simulink model "LQG_tw_v5"  (R2019a)
settings: Solver=FixedStepAuto  StartTime=0.0  StopTime=20  FixedStep=0.01  RelTol=1e-3
undefined symbols (not defined in the file): K
libraries: simulink x3, simulink_extras x2
settings Model: Creator=chute  LastModifiedBy=chute
settings DataIOCC: ReturnWorkspaceOutputs=off

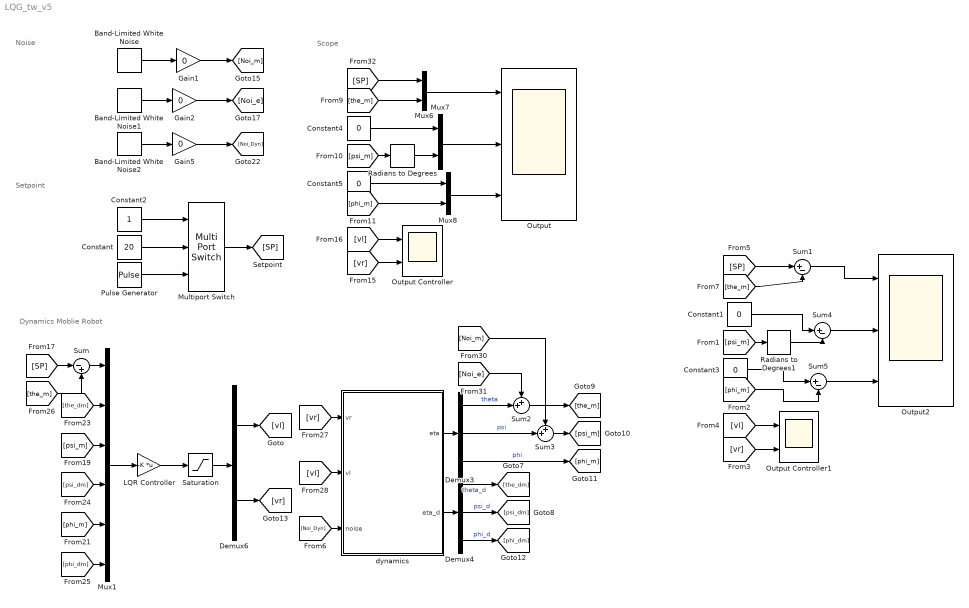
== system LQG_tw_v5 ==
  note: Noise
  note: Scope
  note: Setpoint
  note: Dynamics Moblie Robot
  Band-Limited White Noise : simulink/Sources/Band-Limited White Noise  Cov=[0.0001]  Ts=0.1  seed=[23341]
  Band-Limited White Noise1 : simulink/Sources/Band-Limited White Noise  Cov=[0.0001]  Ts=0.1  seed=[23341]
  Band-Limited White Noise2 : simulink/Sources/Band-Limited White Noise  Cov=[0.0001]  Ts=0.1  seed=[23341]
  Constant : Constant  Value=20
  Constant{1,3..5} (4 alike) : Constant  Value=0
  Constant2 : Constant
  Demux3 : Demux  Outputs=3
  Demux4 : Demux  Outputs=3
  Demux6 : Demux  Outputs=2
  Gain1 : Gain  Gain=0
  Gain2 : Gain  Gain=0
  Gain5 : Gain  Gain=0
  LQR Controller : Gain  Gain=-K  Multiplication=Matrix(K*u) (u vector)
  Multiport Switch : MultiPortSwitch  Inputs=2
  Mux1 : Mux  Inputs=6
  Mux6 : Mux  Inputs=2
  Mux7 : Mux  Inputs=2
  Mux8 : Mux  Inputs=2
  Output : Scope  NumInputPorts=3
  Output Controller : Scope  NumInputPorts=2
  Output Controller1 : Scope  NumInputPorts=2
  Output2 : Scope  NumInputPorts=3
  Pulse Generator : DiscretePulseGenerator  PulseType=Time based  Amplitude=20  Period=10  PulseWidth=50
  Radians to Degrees : simulink_extras/Transformations/Radians to Degrees
  Radians to Degrees1 : simulink_extras/Transformations/Radians to Degrees
  Saturation : Saturate  UpperLimit=12  LowerLimit=-12
  Sum : Sum  Inputs=|-+
  Sum1 : Sum  Inputs=|+-
  Sum2 : Sum  Inputs=++|
  Sum3 : Sum  Inputs=++|
  Sum4 : Sum  Inputs=|+-
  Sum5 : Sum  Inputs=|+-
  dynamics : Subsystem
  wires:
  dynamics/1(eta) -> Demux3/1
  Demux4/1 -> [the_dm]  "theta_d"
  dynamics/2(eta_d) -> Demux4/1
  Demux4/3 -> [phi_dm]  "phi_d"
  Demux4/2 -> [psi_dm]  "psi_d"
  Demux6/1 -> [vl]
  LQR Controller/1 -> Saturation/1
  Mux1/1 -> LQR Controller/1
  Sum/1 -> Mux1/1
  Multiport Switch/1 -> [SP]
  Constant/1 -> Multiport Switch/2
  Constant2/1 -> Multiport Switch/1
  [phi_m] -> Mux1/5
  [psi_m] -> Mux1/3
  [the_dm] -> Mux1/2
  [psi_dm] -> Mux1/4
  [phi_dm] -> Mux1/6
  Band-Limited White Noise/1 -> Gain1/1
  Demux3/3 -> [phi_m]  "phi"
  Sum3/1 -> [psi_m]
  Demux3/2 -> Sum3/2  "psi"
  Demux3/1 -> Sum2/2  "theta"
  Band-Limited White Noise1/1 -> Gain2/1
  [the_m] -> Sum/2
  [vl] -> dynamics/2("vl ")
  [vr] -> dynamics/1(vr)
  Gain1/1 -> [Noi_m]
  Gain2/1 -> [Noi_e]
  [Noi_m] -> Sum3/1
  [Noi_e] -> Sum2/1
  Mux8/1 -> Output/3
  Mux7/1 -> Output/2
  Mux6/1 -> Output/1
  [the_m] -> Mux6/2
  [SP] -> Mux6/1
  [psi_m] -> Radians to Degrees/1
  Constant4/1 -> Mux7/1
  [phi_m] -> Mux8/2
  Constant5/1 -> Mux8/1
  Sum2/1 -> [the_m]
  Demux6/2 -> [vr]
  [SP] -> Sum/1
  Pulse Generator/1 -> Multiport Switch/3
  Gain5/1 -> [Noi_Dyn]
  Band-Limited White Noise2/1 -> Gain5/1
  [Noi_Dyn] -> dynamics/3(noise)
  Saturation/1 -> Demux6/1
  Radians to Degrees/1 -> Mux7/2
  [vl] -> Output Controller/1
  [vr] -> Output Controller/2
  Constant3/1 -> Sum5/1
  Radians to Degrees1/1 -> Sum4/2
  [vl] -> Output Controller1/1
  [the_m] -> Sum1/2
  Constant1/1 -> Sum4/1
  Sum1/1 -> Output2/1
  Sum5/1 -> Output2/3
  [phi_m] -> Sum5/2
  [vr] -> Output Controller1/2
  Sum4/1 -> Output2/2
  [SP] -> Sum1/1
  [psi_m] -> Radians to Degrees1/1

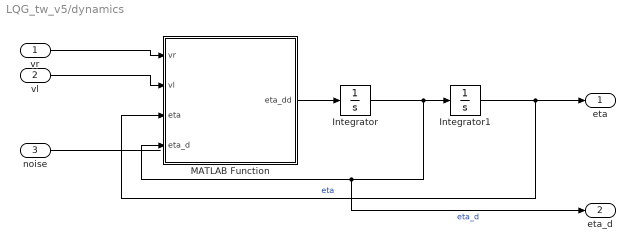
== system LQG_tw_v5/dynamics ==
  vr : Inport
  "vl " : Inport  Port=2
  noise : Inport  Port=3
  Integrator : Integrator  InitialCondition=[0;0;0]
  Integrator1 : Integrator  InitialCondition=[0;0.3*pi/180;0]
  MATLAB Function : MATLAB Function  TreatAsAtomicUnit=on
  eta : Outport
  eta_d : Outport  Port=2
  wires:
  Integrator/1 -> Integrator1/1, eta_d/1, MATLAB Function/4(eta_d)  "eta_d"
  Integrator1/1 -> eta/1, MATLAB Function/3(eta)  "eta"
  MATLAB Function/1(eta_dd) -> Integrator/1
  vr/1 -> MATLAB Function/1(vr)
  "vl "/1 -> MATLAB Function/2(vl)
  noise/1 -> ?

== matlab function LQG_tw_v5/dynamics/MATLAB Function ==
  data: vr input; vl input; eta_dd output; eta input; eta_d input
function eta_dd= fcn(vr,vl,eta,eta_d)
%% declare the parameter:
%% Hoang

g =9.81; % gravity acceleration
m =0.04; % wheel weight
R =0.0325; % Wheel radius
M =0.8;  % body weight
W =0.17; % Body width
D =0.098; % Body depth
H =0.121;% Body Height
L =0.0628;% distance

n =30 ; %gear ratio
Rm=8.0013;      %dien tro dong co DC
Kb=5.9233e-07;   %he so emf cua dong co
Kt=0.023385;   %momemt xoan cua dong co DC\
fm = 0.0022; % friction cof between body and DC motor.
fw = 0.0000001; % friction cof between wheel and floor
anp = (n*Kt)/Rm;
bet = (n*Kt*Kb/Rm)+fm;

J_psi  = M*L^2/3; % Body inertia moment
Jw = m*R^2/2;  %Wheel inertia moment
J_phi = M*(W^2+D^2)/12; % Body yaw inertia moment
Jm = 1.175e-05;
anp = (n*Kt)/Rm;
bet = (n*Kt*Kb/Rm)+fm;




%% Notation:
the=eta(1,1);
psi=eta(2,1);
phi=eta(3,1);

the_dot=eta_d(1,1);
psi_dot=eta_d(2,1);
phi_dot=eta_d(3,1);

tor=[vl;vr];



%% DC Motor
F_the = anp*(vl+vr)-2*(bet+fw)*the_dot+2*bet*psi_dot;
F_psi = -anp*(vl+vr)+2*bet*the_dot-2*bet*psi_dot;
F_phi = W*anp*(vr-vl)/(2*R)-W^2*((bet+fw)*phi_dot)/2*R^2;
tor =[F_the;F_psi;F_phi];

%% dyn
% Mass matrix:
M1 = ...
[2*Jw + 2*Jm*n^2 + R^2*(M + 2*m),L*M*R*cos(psi) - 2*Jm*n^2,0;
 L*M*R*cos(psi) - 2*Jm*n^2,J_psi + L^2*M + 2*Jm*n^2,0;
 0,0,J_phi + (W^2*m)/2 + L^2*M*sin(psi)^2 + (W^2*(Jw + Jm*n^2))/(2*R^2)];

%Coriolis matrix:
C1 = ...
[0,-L*M*R*psi_dot*sin(psi),0;
 0,0,-(L^2*M*phi_dot*sin(2*psi))/2;
 0,(L^2*M*phi_dot*sin(2*psi))/2,(L^2*M*psi_dot*sin(2*psi))/2];


% Gravity vector:
G1=...
[0;
-L*M*g*sin(psi);
0];
%% Input Matrices:
% B1=[1/R,        1/R;
%     -1,          -1;
%     W/(2*R),-W/(2*R)];

%% External Force

eta_dd=inv(M1)*(tor-C1*eta_d-G1);
end
